simulink model "SimuNL"  (R2018a)
settings: Solver=ode45  StartTime=0.0  StopTime=Tsim  RelTol=1e-3  EnableMultiTasking=on
values from neighbouring files (symbols this model uses):
  K1nl = 10    [n_mpc.m]    (also in test_plant.m)
  K2nl = 10    [n_mpc.m]    (also in test_plant.m)
  Qnl = 0.03333    [n_mpc.m]    (also in test_plant.m)
  Vnl = 1    [n_mpc.m]    (also in test_plant.m)
settings Model: Creator=Thiago  LastModifiedBy=marcus
settings SolverCC: AlgebraicLoopSolver=LineSearch
settings DataIOCC: LimitDataPoints=on  SaveFormat=Array
settings OptimizationCC: LifeSpan=inf
settings DebuggingCC: SFUnexpectedBacktrackingDiag=warning  SFNoUnconditionalDefaultTransitionDiag=warning  SFExecutionAtInitializationDiag=none
settings HardwareCC: ProdBitPerPointer=32  ProdBitPerSizeT=32  ProdBitPerPtrDiffT=32  ProdLargestAtomicFloat=None  ProdIntDivRoundTo=Undefined  ProdEndianess=Unspecified  ProdWordSize=32  ProdHWDeviceType=32-bit Generic
settings ModelReferenceCC: PropagateSignalLabelsOutOfModel=off
settings CodeAppCC: StateflowObjectComments=on
settings GRTTargetCC: TargetLangStandard=C89/C90 (ANSI)  GeneratePreprocessorConditionals=Disable all
settings ConfigComp: CovMetricSettings=dw  CovHtmlReporting=on  CovSaveCumulativeToWorkspaceVar=on  CovSaveSingleToWorkspaceVar=on  CovExternalEMLEnable=off

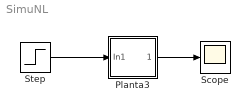
== system SimuNL ==
  " Planta3" : Subsystem
  Scope : Scope
  Step : Step  SampleTime=0
  wires:
  Step/1 -> " Planta3"/1(In1)
  " Planta3"/1(Out1) -> Scope/1

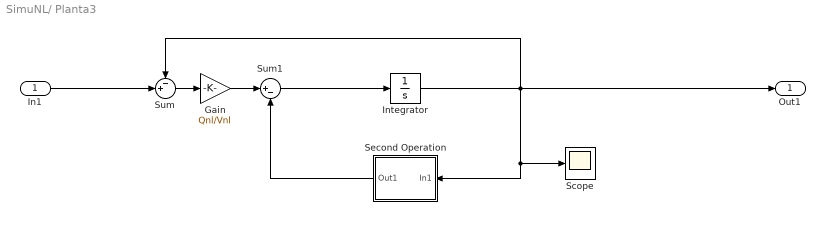
== system SimuNL/ Planta3 ==
  In1 : Inport
  Gain : Gain  Gain=Qnl/Vnl
  Integrator : Integrator  InitialCondition=1
  Scope : Scope
  "Second Operation " : Subsystem
  Sum : Sum  Inputs=-+|
  Sum1 : Sum  Inputs=|+-
  Out1 : Outport
  wires:
  Integrator/1 -> Out1/1, Sum/1, "Second Operation "/1(In1), Scope/1
  In1/1 -> Sum/2
  Sum1/1 -> Integrator/1
  "Second Operation "/1(Out1) -> Sum1/2
  Gain/1 -> Sum1/1
  Sum/1 -> Gain/1

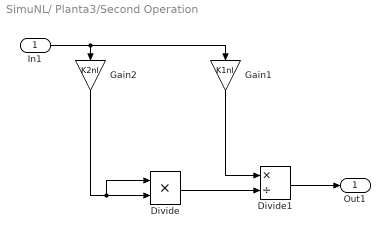
== system SimuNL/ Planta3/Second Operation  ==
  In1 : Inport
  Divide : Product  Inputs=**
  Divide1 : Product  Inputs=*/
  Gain1 : Gain  Gain=K1nl
  Gain2 : Gain  Gain=K2nl
  Out1 : Outport
  wires:
  In1/1 -> Gain2/1, Gain1/1
  Divide1/1 -> Out1/1
  Divide/1 -> Divide1/2
  Gain1/1 -> Divide1/1
  Gain2/1 -> Divide/2, Divide/1
